simulink model "lab3"  (R2021a)
settings: Solver=VariableStepDiscrete  StartTime=0.0  StopTime=2e-3  RelTol=1e-3
libraries: dspsrcs4 x4, commseqgen3 x3, dsparch4 x2, commutil2 x2, commchan3 x1
settings Model: Creator=Tomas  LastModifiedBy=Tomas

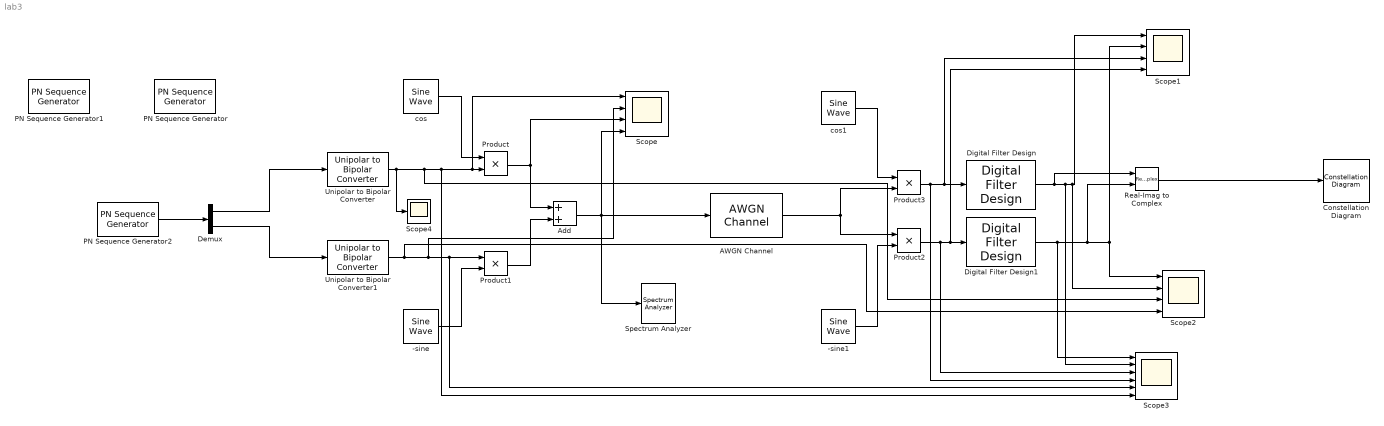
== system lab3 ==
  -sine : dspsrcs4/Sine Wave  Amplitude=1  Frequency=40e6  Phase=pi  SampleMode=Discrete  OutComplex=Real  CompMethod=Trigonometric fcn  TableSize=Speed  SampleTime=1/400e6  SamplesPerFrame=1  ResetState=Restart at time zero  OutputFrames=off  dataType=double  wordLen=16  udDataType=sfix(16)  fracBitsMode=Best precision  numFracBits=15  OutDataTypeStr=double  LastOutDataTypeStr=double
  -sine1 : dspsrcs4/Sine Wave  Amplitude=1  Frequency=40e6  Phase=pi  SampleMode=Discrete  OutComplex=Real  CompMethod=Trigonometric fcn  TableSize=Speed  SampleTime=1/400e6  SamplesPerFrame=1  ResetState=Restart at time zero  OutputFrames=off  dataType=double  wordLen=16  udDataType=sfix(16)  fracBitsMode=Best precision  numFracBits=15  OutDataTypeStr=double  LastOutDataTypeStr=double
  AWGN Channel : commchan3/AWGN Channel  InputProcessing=Columns as channels (frame based)  seed=67  noiseMode="Signal to noise ratio  (Eb/No)"  EbNodB=200  EsNodB=10  SNRdB=30  bitsPerSym=2  Ps=1  Tsym=1/500e3  variance=1
  Add : Sum
  Constellation Diagram : ConstellationDiagram
  Demux : Demux  Outputs=2
  Digital Filter Design : dsparch4/Digital Filter Design  mwdsp_browser_bugfix_var=off
  Digital Filter Design1 : dsparch4/Digital Filter Design  mwdsp_browser_bugfix_var=off
  PN Sequence Generator : commseqgen3/PN Sequence Generator  poly='z^7+z^6+1'  ini_sta=[1 1 1 1 1 1 1]  outBitMaskSource=Dialog parameter  shift=0  outVarSiz=off  maxOutSizeMode=Dialog parameter  maxOutSize=[10 1]  Ts=1/500e3  sampPerFrame=1  reset=off  bitPackedOutputs=off  outDataType=double  numPackedBits=8  bitPackDataSigned=off  bitPackedOutDType=double
  PN Sequence Generator1 : commseqgen3/PN Sequence Generator  poly='z^7 + z^6 + 1'  ini_sta=[1 1 1 0 0 0 1]  outBitMaskSource=Dialog parameter  shift=0  outVarSiz=off  maxOutSizeMode=Dialog parameter  maxOutSize=[10 1]  Ts=1/500e3  sampPerFrame=1  reset=off  bitPackedOutputs=off  outDataType=double  numPackedBits=8  bitPackDataSigned=off  bitPackedOutDType=double
  PN Sequence Generator2 : commseqgen3/PN Sequence Generator  poly='z^7+z^6+1'  ini_sta=[1 1 1 1 1 1 1]  outBitMaskSource=Dialog parameter  shift=0  outVarSiz=off  maxOutSizeMode=Dialog parameter  maxOutSize=[10 1]  Ts=1/1e6  sampPerFrame=2  reset=off  bitPackedOutputs=off  outDataType=double  numPackedBits=8  bitPackDataSigned=off  bitPackedOutDType=double
  Product{,1..3} (4 alike) : Product
  Real-Imag to Complex : RealImagToComplex  SampleTime=1/500e3
  Scope : Scope  NumInputPorts=4
  Scope1 : Scope  NumInputPorts=4
  Scope2 : Scope  NumInputPorts=4
  Scope3 : Scope  NumInputPorts=6
  Scope4 : Scope
  Spectrum Analyzer : SpectrumAnalyzer
  Unipolar to Bipolar Converter : commutil2/Unipolar to Bipolar Converter  M=2  polarity=Positive  dataType=Inherit via internal rule
  Unipolar to Bipolar Converter1 : commutil2/Unipolar to Bipolar Converter  M=2  polarity=Positive  dataType=Inherit via internal rule
  cos : dspsrcs4/Sine Wave  Amplitude=1  Frequency=40e6  Phase=pi/2  SampleMode=Discrete  OutComplex=Real  CompMethod=Trigonometric fcn  TableSize=Speed  SampleTime=1/400e6  SamplesPerFrame=1  ResetState=Restart at time zero  OutputFrames=off  dataType=double  wordLen=16  udDataType=sfix(16)  fracBitsMode=Best precision  numFracBits=15  OutDataTypeStr=double  LastOutDataTypeStr=double
  cos1 : dspsrcs4/Sine Wave  Amplitude=1  Frequency=40e6  Phase=pi/2  SampleMode=Discrete  OutComplex=Real  CompMethod=Trigonometric fcn  TableSize=Speed  SampleTime=1/400e6  SamplesPerFrame=1  ResetState=Restart at time zero  OutputFrames=off  dataType=double  wordLen=16  udDataType=sfix(16)  fracBitsMode=Best precision  numFracBits=15  OutDataTypeStr=double  LastOutDataTypeStr=double
  wires:
  -sine/1 -> Product1/2
  cos/1 -> Product/1
  Unipolar to Bipolar Converter/1 -> Scope4/1, Scope2/3, Scope3/6, Scope/1, Product/2
  Unipolar to Bipolar Converter1/1 -> Scope2/4, Scope3/5, Product1/1, Scope/2
  Product/1 -> Scope/3, Add/1
  Product1/1 -> Add/2
  Add/1 -> AWGN Channel/1, Scope/4, Spectrum Analyzer/1
  cos1/1 -> Product3/1
  -sine1/1 -> Product2/2
  AWGN Channel/1 -> Product3/2, Product2/1
  Product3/1 -> Scope3/4, Scope1/3, Digital Filter Design/1
  Product2/1 -> Scope3/3, Scope1/4, Digital Filter Design1/1
  Digital Filter Design/1 -> Real-Imag to Complex/1, Scope3/2, Scope2/2, Scope1/1
  Digital Filter Design1/1 -> Scope3/1, Real-Imag to Complex/2, Scope2/1, Scope1/2
  PN Sequence Generator2/1 -> Demux/1
  Demux/1 -> Unipolar to Bipolar Converter/1
  Demux/2 -> Unipolar to Bipolar Converter1/1
  Real-Imag to Complex/1 -> Constellation Diagram/1
